simulink model "multiportswitch_test"  (Simulink 8.4)
settings: Solver=VariableStepDiscrete  StartTime=0.0  StopTime=0  MaxStep=1  RelTol=1e-3
settings Model: Creator=arnaud  LastModifiedBy=arnaud
settings DataIOCC: SaveFormat=Structure  SignalLoggingSaveFormat=Dataset
settings OptimizationCC: ExpressionDepthLimit=128
settings DebuggingCC: UnderspecifiedInitializationDetection=Simplified  MergeDetectMultiDrivingBlocksExec=error  FcnCallInpInsideContextMsg=EnableAllAsError  StateNameClashWarn=none
settings GRTTargetCC: CombineOutputUpdateFcns=on  GRTInterface=off

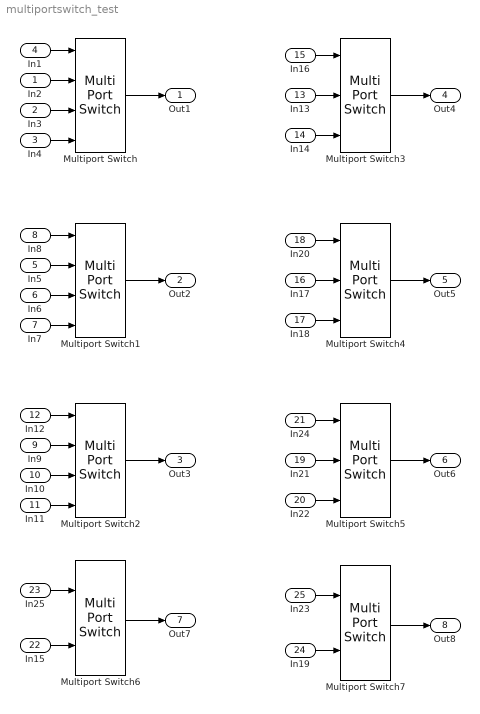
== system multiportswitch_test ==
  In2 : Inport  PortDimensions=[2 3]
  In3 : Inport  Port=2
  In4 : Inport  Port=3  PortDimensions=[2 3]
  In1 : Inport  Port=4  OutDataTypeStr=int8  PortDimensions=[2 3]
  In5 : Inport  Port=5  PortDimensions=1
  In6 : Inport  Port=6  PortDimensions=1
  In7 : Inport  Port=7  PortDimensions=1
  In8 : Inport  Port=8  OutDataTypeStr=int8  PortDimensions=1
  In9 : Inport  Port=9  PortDimensions=1
  In10 : Inport  Port=10  PortDimensions=1
  In11 : Inport  Port=11  PortDimensions=1
  In12 : Inport  Port=12  OutDataTypeStr=int8  PortDimensions=1
  In13 : Inport  Port=13  PortDimensions=[2 3]
  In14 : Inport  Port=14
  In16 : Inport  Port=15  OutDataTypeStr=int8  PortDimensions=[2 3]
  In17 : Inport  Port=16  PortDimensions=1
  In18 : Inport  Port=17  PortDimensions=1
  In20 : Inport  Port=18  OutDataTypeStr=int8  PortDimensions=1
  In21 : Inport  Port=19  PortDimensions=1
  In22 : Inport  Port=20  PortDimensions=1
  In24 : Inport  Port=21  OutDataTypeStr=int8  PortDimensions=1
  In15 : Inport  Port=22  PortDimensions=1
  In25 : Inport  Port=23  OutDataTypeStr=int8  PortDimensions=1
  In19 : Inport  Port=24  PortDimensions=3
  In23 : Inport  Port=25  OutDataTypeStr=int8  PortDimensions=1
  Multiport Switch : MultiPortSwitch  DataPortOrder=Specify indices  DataPortIndices={1,[2,3]}  DataPortForDefault=Additional data port  DiagnosticForDefault=Warning
  Multiport Switch1 : MultiPortSwitch  DataPortOrder=Zero-based contiguous  Inputs=2  DataPortIndices={1,[2,3]}  DataPortForDefault=Additional data port  DiagnosticForDefault=Warning
  Multiport Switch2 : MultiPortSwitch  Inputs=2  DataPortIndices={1,[2,3]}  DataPortForDefault=Additional data port  DiagnosticForDefault=Warning
  Multiport Switch3 : MultiPortSwitch  DataPortOrder=Specify indices  DataPortIndices={1,[2,3]}  DiagnosticForDefault=Warning
  Multiport Switch4 : MultiPortSwitch  DataPortOrder=Zero-based contiguous  Inputs=2  DataPortIndices={1,[2,3]}  DiagnosticForDefault=Warning
  Multiport Switch5 : MultiPortSwitch  Inputs=2  DataPortIndices={1,[2,3]}  DiagnosticForDefault=Warning
  Multiport Switch6 : MultiPortSwitch  DataPortOrder=Zero-based contiguous  Inputs=1  DataPortIndices={1,[2,3]}  DataPortForDefault=Additional data port  DiagnosticForDefault=Warning
  Multiport Switch7 : MultiPortSwitch  DataPortOrder=Zero-based contiguous  Inputs=1  DataPortIndices={[1,2,3]}  DataPortForDefault=Additional data port  DiagnosticForDefault=Warning  OutDataTypeStr=Inherit: Inherit via back propagation
  Out1 : Outport
  Out2 : Outport  Port=2
  Out3 : Outport  Port=3
  Out4 : Outport  Port=4
  Out5 : Outport  Port=5
  Out6 : Outport  Port=6
  Out7 : Outport  Port=7
  Out8 : Outport  Port=8
  wires:
  Multiport Switch/1 -> Out1/1
  In2/1 -> Multiport Switch/2
  In3/1 -> Multiport Switch/3
  In4/1 -> Multiport Switch/4
  In1/1 -> Multiport Switch/1
  Multiport Switch1/1 -> Out2/1
  In5/1 -> Multiport Switch1/2
  In6/1 -> Multiport Switch1/3
  In7/1 -> Multiport Switch1/4
  In8/1 -> Multiport Switch1/1
  Multiport Switch2/1 -> Out3/1
  In9/1 -> Multiport Switch2/2
  In10/1 -> Multiport Switch2/3
  In11/1 -> Multiport Switch2/4
  In12/1 -> Multiport Switch2/1
  Multiport Switch3/1 -> Out4/1
  In13/1 -> Multiport Switch3/2
  In14/1 -> Multiport Switch3/3
  In16/1 -> Multiport Switch3/1
  Multiport Switch4/1 -> Out5/1
  In17/1 -> Multiport Switch4/2
  In18/1 -> Multiport Switch4/3
  In20/1 -> Multiport Switch4/1
  Multiport Switch5/1 -> Out6/1
  In21/1 -> Multiport Switch5/2
  In22/1 -> Multiport Switch5/3
  In24/1 -> Multiport Switch5/1
  Multiport Switch6/1 -> Out7/1
  In15/1 -> Multiport Switch6/2
  In25/1 -> Multiport Switch6/1
  Multiport Switch7/1 -> Out8/1
  In19/1 -> Multiport Switch7/2
  In23/1 -> Multiport Switch7/1
